simulink model "controllerSharedMem"  (Simulink 8.0)
settings: Solver=FixedStepDiscrete  StartTime=0.0  StopTime=inf  RelTol=1e-3
InitFcn:
  | initSharedMem;
values from neighbouring files (symbols this model uses):
  k = [  10    0.1   2 ... (first row only)    [initRov14.m]    (also in initSharedMem.m = [ 20    5   15)
  kw = block.InputPort(6).Data    [desiredForceComputation.m]    (also in initBalancingControllerWithHandControl.m = 5; initSharedMem.m = 1; initTorqueBalancing.m = 4; initTorqueBalancingWithNonlinearImpedences.m = 1)
  nc = 12    [initCompleteForceControlSim.m]    (also in initPartialForceControl.m = 6; initPartialForceControlSim.m = 6; initSharedMem.m)
  nj = 25    [initCompleteForceControlSim.m]    (also in initMonitor.m; initMonitorSim.m; initPartialForceControl.m; initPartialForceControlSim.m)
undefined symbols (not defined in the file or in its folder): DiscIntNeverNeededParam
libraries: WBCLibrary x17, simulink x3, dspsigops x3
settings Model: Creator=daniele  LastModifiedBy=makaveli
settings DebuggingCC: FcnCallInpInsideContextMsg=EnableAllAsWarning
settings GRTTargetCC: CombineOutputUpdateFcns=off  GRTInterface=on

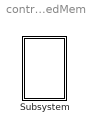
== system controllerSharedMem ==
  Subsystem : Subsystem  mask{robotName='icubGazeboSim', Ts=0.01, localName='dynamicBalancing'}
      mask prompts: robotName "robot name"; localName "module name"

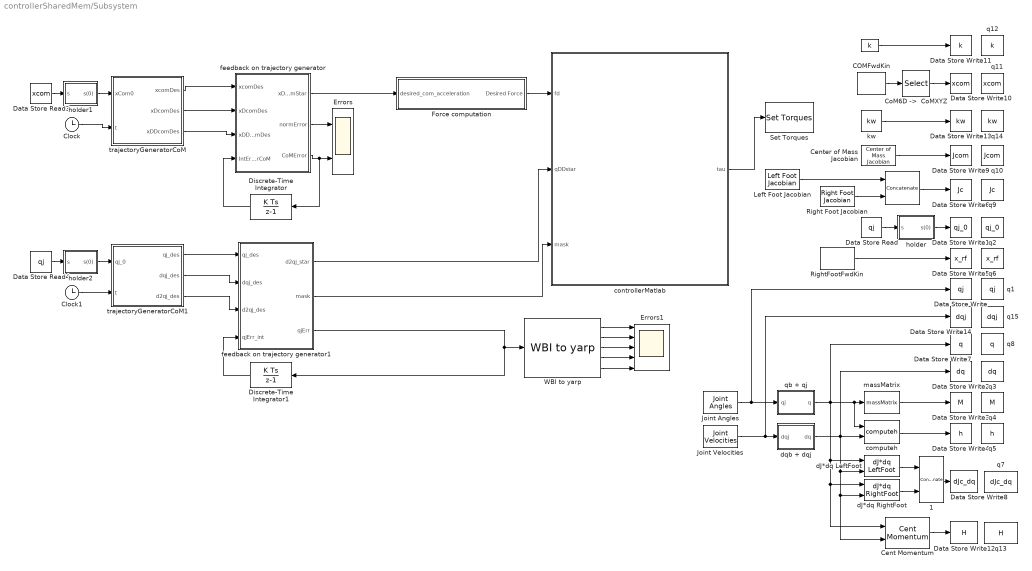
== system controllerSharedMem/Subsystem ==
  "    " : Constant  Value=k
  " " : Concatenate  Mode=Multidimensional array
  " 1" : Concatenate  Mode=Multidimensional array
  "COMFwdKin " : WBCLibrary/wholeBodyModel/Forward Kinematics/COMFwdKin   robotName=robotName  localName=localName
  Cent Momentum : WBCLibrary/wholeBodyModel/Dynamics/Cent Momentum  robotName=robotName  localName=localName
  Center of Mass Jacobian : WBCLibrary/wholeBodyModel/Jacobians/Center of Mass Jacobian  robotName=robotName  localName=localName
  Clock : Clock
  Clock1 : Clock
  "CoM6D ->  CoMXYZ" : Selector  InputPortWidth=7  IndexOptions=Index vector (dialog)  Indices=[1 2 3]  OutputSizes=1
  Data Store Read : DataStoreRead  DataStoreName=qj
  Data Store Read3 : DataStoreRead  DataStoreName=xcom
  Data Store Read4 : DataStoreRead  DataStoreName=qj
  Data Store Write : DataStoreWrite  Priority=-1  DataStoreName=qj
  Data Store Write1 : DataStoreWrite  Priority=-1  DataStoreName=qj_0
  Data Store Write10 : DataStoreWrite  Priority=-1  DataStoreName=xcom
  Data Store Write11 : DataStoreWrite  Priority=-1  DataStoreName=k
  Data Store Write12 : DataStoreWrite  Priority=-1  DataStoreName=H
  Data Store Write13 : DataStoreWrite  Priority=-1  DataStoreName=kw
  Data Store Write14 : DataStoreWrite  Priority=-1  DataStoreName=dqj
  Data Store Write2 : DataStoreWrite  Priority=-1  DataStoreName=dq
  Data Store Write3 : DataStoreWrite  Priority=-1  DataStoreName=M
  Data Store Write4 : DataStoreWrite  Priority=-1  DataStoreName=h
  Data Store Write5 : DataStoreWrite  Priority=-1  DataStoreName=x_rf
  Data Store Write6 : DataStoreWrite  Priority=-1  DataStoreName=Jc
  Data Store Write7 : DataStoreWrite  Priority=-1  DataStoreName=q
  Data Store Write8 : DataStoreWrite  Priority=-1  DataStoreName=dJc_dq
  Data Store Write9 : DataStoreWrite  Priority=-1  DataStoreName=Jcom
  Discrete-Time Integrator : DiscreteIntegrator  InitialCondition=[0;0;0]  SampleTime=Ts  ICPrevOutput=DiscIntNeverNeededParam  ICPrevScaledInput=DiscIntNeverNeededParam
  Discrete-Time Integrator1 : DiscreteIntegrator  InitialCondition=zeros(nj,1)  SampleTime=Ts  ICPrevOutput=DiscIntNeverNeededParam  ICPrevScaledInput=DiscIntNeverNeededParam
  Errors : Scope  NumInputPorts=2
      settings: TimeRange=70  YMin=0~-0.025  YMax=0.0325~0.0325  SaveName=ScopeData6
  Errors1 : Scope  NumInputPorts=5
      settings: TimeRange=70  YMin=-0.2~-0.1~-0.075~-0.25~-0.2  YMax=0.25~0.075~0.1~0.25~0.25
  Force computation : Subsystem
  Joint Angles : WBCLibrary/wholeBodyStates/Joint Angles  robotName=robotName  localName=localName
  Joint Velocities : WBCLibrary/wholeBodyStates/Joint Velocities  robotName=robotName  localName=localName
  Left Foot Jacobian : WBCLibrary/wholeBodyModel/Jacobians/Left Foot Jacobian  robotName=robotName  localName=localName
  Right Foot Jacobian : WBCLibrary/wholeBodyModel/Jacobians/Right Foot Jacobian  robotName=robotName  localName=localName
  RightFootFwdKin : WBCLibrary/wholeBodyModel/Forward Kinematics/RightFootFwdKin  robotName=robotName  localName=localName
  Set Torques : WBCLibrary/wholeBodyActuators/Set Torques  val=6  robotName=robotName  localName=localName
  WBI to yarp : WBCLibrary/Utilities/WBI to yarp
  computeh : WBCLibrary/wholeBodyModel/Dynamics/computeh  val=7  robotname=robotName  localname=localName
  controllerMatlab : MATLAB Function  TreatAsAtomicUnit=on
  dJ*dq LeftFoot : WBCLibrary/wholeBodyModel/Dynamics/dJ*dq LeftFoot  val=9  robotName=robotName  localName=localName
  dJ*dq RightFoot : WBCLibrary/wholeBodyModel/Dynamics/dJ*dq RightFoot  val=9  robotName=robotName  localName=localName
  dqb + dqj : Subsystem
  feedback on trajectory generator : MATLAB Function  TreatAsAtomicUnit=on
  feedback on trajectory generator1 : MATLAB Function  TreatAsAtomicUnit=on
  holder : Subsystem
  holder1 : Subsystem
  holder2 : Subsystem
  kw : Constant  Value=kw
  massMatrix : WBCLibrary/wholeBodyModel/Dynamics/massMatrix  val=8  robotname=robotName  localname=localName
  q1 : DataStoreMemory  Priority=-1  DataStoreName=qj  ReadBeforeWriteMsg=warning  WriteAfterWriteMsg=warning  WriteAfterReadMsg=warning  InitialValue=zeros(nj,1)  VectorParams1D=off  OutDataTypeStr=double
  q10 : DataStoreMemory  Priority=-1  DataStoreName=Jcom  ReadBeforeWriteMsg=warning  WriteAfterWriteMsg=warning  WriteAfterReadMsg=warning  InitialValue=zeros(6,nj+6)  VectorParams1D=off  OutDataTypeStr=double
  q11 : DataStoreMemory  Priority=-1  DataStoreName=xcom  ReadBeforeWriteMsg=warning  WriteAfterWriteMsg=warning  WriteAfterReadMsg=warning  InitialValue=zeros(3,1)  VectorParams1D=off  OutDataTypeStr=double
  q12 : DataStoreMemory  Priority=-1  DataStoreName=k  ReadBeforeWriteMsg=warning  WriteAfterWriteMsg=warning  WriteAfterReadMsg=warning  InitialValue=k  VectorParams1D=off  OutDataTypeStr=double
  q13 : DataStoreMemory  Priority=-1  DataStoreName=H  ReadBeforeWriteMsg=warning  WriteAfterWriteMsg=warning  WriteAfterReadMsg=warning  InitialValue=zeros(6,1)  VectorParams1D=off  OutDataTypeStr=double
  q14 : DataStoreMemory  Priority=-1  DataStoreName=kw  ReadBeforeWriteMsg=warning  WriteAfterWriteMsg=warning  WriteAfterReadMsg=warning  InitialValue=kw  VectorParams1D=off  OutDataTypeStr=double
  q15 : DataStoreMemory  Priority=-1  DataStoreName=dqj  ReadBeforeWriteMsg=warning  WriteAfterWriteMsg=warning  WriteAfterReadMsg=warning  InitialValue=zeros(nj,1)  VectorParams1D=off  OutDataTypeStr=double
  q2 : DataStoreMemory  Priority=-1  DataStoreName=qj_0  ReadBeforeWriteMsg=warning  WriteAfterWriteMsg=warning  WriteAfterReadMsg=warning  InitialValue=zeros(nj,1)  VectorParams1D=off  OutDataTypeStr=double
  q3 : DataStoreMemory  Priority=-1  DataStoreName=dq  ReadBeforeWriteMsg=warning  WriteAfterWriteMsg=warning  WriteAfterReadMsg=warning  InitialValue=zeros(nj+6,1)  VectorParams1D=off  OutDataTypeStr=double
  q4 : DataStoreMemory  Priority=-1  DataStoreName=M  ReadBeforeWriteMsg=warning  WriteAfterWriteMsg=warning  WriteAfterReadMsg=warning  InitialValue=zeros(nj+6,nj+6)  VectorParams1D=off  OutDataTypeStr=double
  q5 : DataStoreMemory  Priority=-1  DataStoreName=h  ReadBeforeWriteMsg=warning  WriteAfterWriteMsg=warning  WriteAfterReadMsg=warning  InitialValue=zeros(nj+6,1)  VectorParams1D=off  OutDataTypeStr=double
  q6 : DataStoreMemory  Priority=-1  DataStoreName=x_rf  ReadBeforeWriteMsg=warning  WriteAfterWriteMsg=warning  WriteAfterReadMsg=warning  InitialValue=zeros(7,1)  VectorParams1D=off  OutDataTypeStr=double
  q7 : DataStoreMemory  Priority=-1  DataStoreName=dJc_dq  ReadBeforeWriteMsg=warning  WriteAfterWriteMsg=warning  WriteAfterReadMsg=warning  InitialValue=zeros(nc,1)  VectorParams1D=off  OutDataTypeStr=double
  q8 : DataStoreMemory  Priority=-1  DataStoreName=q  ReadBeforeWriteMsg=warning  WriteAfterWriteMsg=warning  WriteAfterReadMsg=warning  InitialValue=zeros(nj+16,1)  VectorParams1D=off  OutDataTypeStr=double
  q9 : DataStoreMemory  Priority=-1  DataStoreName=Jc  ReadBeforeWriteMsg=warning  WriteAfterWriteMsg=warning  WriteAfterReadMsg=warning  InitialValue=zeros(nc,nj+6)  VectorParams1D=off  OutDataTypeStr=double
  qb + qj : Subsystem
  trajectoryGeneratorCoM : MATLAB Function  TreatAsAtomicUnit=on
  trajectoryGeneratorCoM1 : MATLAB Function  TreatAsAtomicUnit=on
  wires:
  Left Foot Jacobian/1 -> " "/1
  Right Foot Jacobian/1 -> " "/2
  qb + qj/1(q) -> massMatrix/1, computeh/1, dJ*dq LeftFoot/1, Cent Momentum/1, dJ*dq RightFoot/1, Data Store Write7/1
  dqb + dqj/1(dq) -> computeh/2, dJ*dq LeftFoot/2, Cent Momentum/2, dJ*dq RightFoot/2, Data Store Write2/1
  Data Store Read/1 -> holder/1(s)
  holder/1(s(0)) -> Data Store Write1/1
  massMatrix/1 -> Data Store Write3/1
  computeh/1 -> Data Store Write4/1
  Joint Velocities/1 -> dqb + dqj/1(dqj), Data Store Write14/1
  RightFootFwdKin/1 -> Data Store Write5/1
  " "/1 -> Data Store Write6/1
  "    "/1 -> Data Store Write11/1
  Center of Mass Jacobian/1 -> Data Store Write9/1
  "COMFwdKin "/1 -> "CoM6D ->  CoMXYZ"/1
  "CoM6D ->  CoMXYZ"/1 -> Data Store Write10/1
  Clock/1 -> trajectoryGeneratorCoM/2(t)
  holder1/1(s(0)) -> trajectoryGeneratorCoM/1(xCom0)
  dJ*dq LeftFoot/1 -> " 1"/1
  dJ*dq RightFoot/1 -> " 1"/2
  " 1"/1 -> Data Store Write8/1
  Cent Momentum/1 -> Data Store Write12/1
  kw/1 -> Data Store Write13/1
  controllerMatlab/1(tau) -> Set Torques/1
  Data Store Read3/1 -> holder1/1(s)
  trajectoryGeneratorCoM/1(xcomDes) -> feedback on trajectory generator/1(xcomDes)
  trajectoryGeneratorCoM/2(xDcomDes) -> feedback on trajectory generator/2(xDcomDes)
  trajectoryGeneratorCoM/3(xDDcomDes) -> feedback on trajectory generator/3(xDDcomDes)
  Discrete-Time Integrator/1 -> feedback on trajectory generator/4(IntErrorCoM)
  feedback on trajectory generator/2(normError) -> Errors/1
  Clock1/1 -> trajectoryGeneratorCoM1/2(t)
  holder2/1(s(0)) -> trajectoryGeneratorCoM1/1(qj_0)
  Data Store Read4/1 -> holder2/1(s)
  trajectoryGeneratorCoM1/1(qj_des) -> feedback on trajectory generator1/1(qj_des)
  trajectoryGeneratorCoM1/2(dqj_des) -> feedback on trajectory generator1/2(dqj_des)
  trajectoryGeneratorCoM1/3(d2qj_des) -> feedback on trajectory generator1/3(d2qj_des)
  Discrete-Time Integrator1/1 -> feedback on trajectory generator1/4(qjErr_int)
  Joint Angles/1 -> qb + qj/1(qj), Data Store Write/1
  feedback on trajectory generator/3(CoMError) -> Errors/2, Discrete-Time Integrator/1
  feedback on trajectory generator1/1(d2qj_star) -> controllerMatlab/2(qDDstar)
  WBI to yarp/1 -> Errors1/1
  WBI to yarp/2 -> Errors1/2
  WBI to yarp/3 -> Errors1/3
  WBI to yarp/4 -> Errors1/4
  WBI to yarp/5 -> Errors1/5
  feedback on trajectory generator1/3(qjErr) -> WBI to yarp/1, Discrete-Time Integrator1/1
  feedback on trajectory generator1/2(mask) -> controllerMatlab/3(mask)
  feedback on trajectory generator/1(xDDcomStar) -> Force computation/1(desired_com_acceleration)
  Force computation/1(Desired Force) -> controllerMatlab/1(fd)

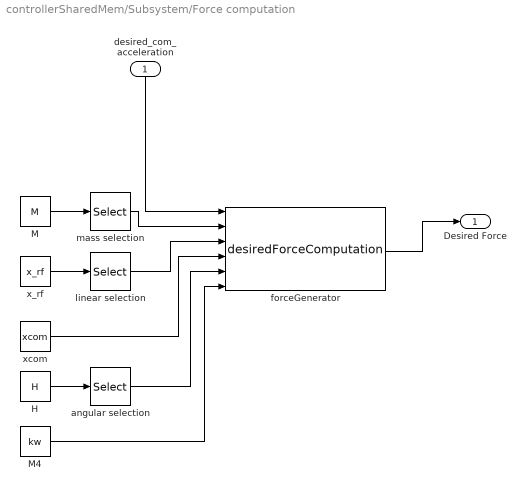
== system controllerSharedMem/Subsystem/Force computation ==
  desired_com_acceleration : Inport
  H : DataStoreRead  DataStoreName=H
  M : DataStoreRead  DataStoreName=M
  M4 : DataStoreRead  DataStoreName=kw
  angular selection : Selector  InputPortWidth=6  IndexOptions=Index vector (dialog)  Indices=[4:6]  OutputSizes=1
  forceGenerator : M-S-Function  FunctionName=desiredForceComputation
  linear selection : Selector  InputPortWidth=7  IndexOptions=Index vector (dialog)  Indices=[1:3]  OutputSizes=1
  mass selection : Selector  NumberOfDimensions=2  InputPortWidth=3  IndexOptions=Index vector (dialog),Index vector (dialog)  Indices=1,1  OutputSizes=1,1
  x_rf : DataStoreRead  DataStoreName=x_rf
  xcom : DataStoreRead  DataStoreName=xcom
  Desired Force : Outport
  wires:
  forceGenerator/1 -> Desired Force/1
  mass selection/1 -> forceGenerator/2
  x_rf/1 -> linear selection/1
  xcom/1 -> forceGenerator/4
  desired_com_acceleration/1 -> forceGenerator/1
  M/1 -> mass selection/1
  linear selection/1 -> forceGenerator/3
  angular selection/1 -> forceGenerator/5
  H/1 -> angular selection/1
  M4/1 -> forceGenerator/6

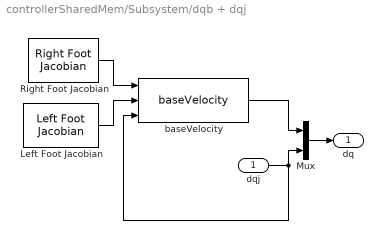
== system controllerSharedMem/Subsystem/dqb + dqj ==
  dqj : Inport
  Left Foot Jacobian : WBCLibrary/wholeBodyModel/Jacobians/Left Foot Jacobian  robotName=robotName  localName=localName
  Mux : Mux  Inputs=2
  Right Foot Jacobian : WBCLibrary/wholeBodyModel/Jacobians/Right Foot Jacobian  robotName=robotName  localName=localName
  baseVelocity : WBCLibrary/Utilities/baseVelocity
  dq : Outport
  wires:
  Left Foot Jacobian/1 -> baseVelocity/2
  Right Foot Jacobian/1 -> baseVelocity/1
  baseVelocity/1 -> Mux/1
  dqj/1 -> baseVelocity/3, Mux/2
  Mux/1 -> dq/1

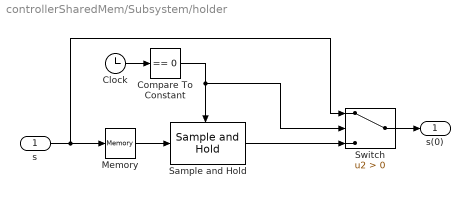
== system controllerSharedMem/Subsystem/holder ==
  s : Inport
  Clock : Clock
  Compare To Constant : simulink/Logic and Bit Operations/Compare To Constant  relop===  const=0  OutDataTypeStr=boolean
  Memory : Memory
  Sample and Hold : dspsigops/Sample and Hold  trig=Falling edge  initCond=0  latchinput=off
  Switch : Switch  Criteria=u2 > Threshold
  s(0) : Outport
  wires:
  s/1 -> Switch/1, Memory/1
  Clock/1 -> Compare To Constant/1
  Compare To Constant/1 -> Sample and Hold/Trigger, Switch/2
  Sample and Hold/1 -> Switch/3
  Switch/1 -> s(0)/1
  Memory/1 -> Sample and Hold/1

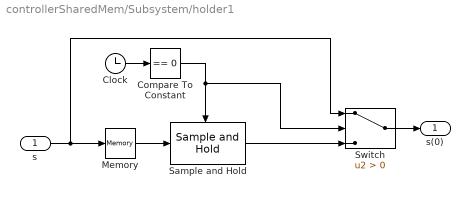
== system controllerSharedMem/Subsystem/holder1 ==
  s : Inport
  Clock : Clock
  Compare To Constant : simulink/Logic and Bit Operations/Compare To Constant  relop===  const=0  OutDataTypeStr=boolean
  Memory : Memory
  Sample and Hold : dspsigops/Sample and Hold  trig=Falling edge  initCond=0  latchinput=off
  Switch : Switch  Criteria=u2 > Threshold
  s(0) : Outport
  wires:
  s/1 -> Switch/1, Memory/1
  Clock/1 -> Compare To Constant/1
  Compare To Constant/1 -> Sample and Hold/Trigger, Switch/2
  Sample and Hold/1 -> Switch/3
  Switch/1 -> s(0)/1
  Memory/1 -> Sample and Hold/1

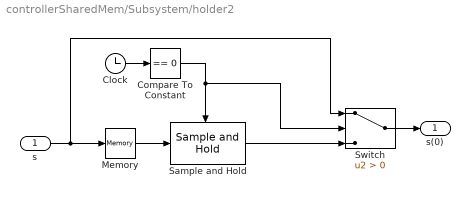
== system controllerSharedMem/Subsystem/holder2 ==
  s : Inport
  Clock : Clock
  Compare To Constant : simulink/Logic and Bit Operations/Compare To Constant  relop===  const=0  OutDataTypeStr=boolean
  Memory : Memory
  Sample and Hold : dspsigops/Sample and Hold  trig=Falling edge  initCond=0  latchinput=off
  Switch : Switch  Criteria=u2 > Threshold
  s(0) : Outport
  wires:
  s/1 -> Switch/1, Memory/1
  Clock/1 -> Compare To Constant/1
  Compare To Constant/1 -> Sample and Hold/Trigger, Switch/2
  Sample and Hold/1 -> Switch/3
  Switch/1 -> s(0)/1
  Memory/1 -> Sample and Hold/1

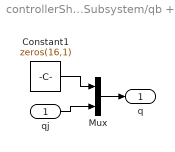
== system controllerSharedMem/Subsystem/qb + qj ==
  qj : Inport
  Constant1 : Constant  Value=zeros(16,1)
  Mux : Mux  Inputs=2
  q : Outport
  wires:
  Mux/1 -> q/1
  Constant1/1 -> Mux/1
  qj/1 -> Mux/2

== matlab function Subsystem/trajectoryGeneratorCoM ==
  data: xcomDes output double; xCom0 input double; t input double; Jcom data_store_memory double; xDcomDes output double; xDDcomDes output double; dq data_store_memory double; k data_store_memory double
function [xcomDes, xDcomDes, xDDcomDes]  = trajGen(xCom0,t)
%#codegen


e3 = [0;1;0];
A = 0.1;
f = 0.1;
t = t*0.8;
% xcomDes    = [xCom0(1:2); (1/A-1)*A*xCom0(3)] + A*xCom0(3)*cos(2*pi*f*t)*e3;
% xDcomDes   = -xCom0(3)*A*2*pi*f*sin(2*pi*f*t)*e3;
% xDDcomDes  = -xCom0(3)*A*(2*pi*f)^2*cos(2*pi*f*t)*e3;

xcomDes    = xCom0 + A*sin(2*pi*f*t)*e3;
xDcomDes   =         A*2*pi*f*cos(2*pi*f*t)*e3;
xDDcomDes  =        -A*(2*pi*f)^2*sin(2*pi*f*t)*e3;

== matlab function Subsystem/controllerMatlab ==
  data: qj data_store_memory double; qj_0 data_store_memory double; dq data_store_memory double; M data_store_memory double; h data_store_memory double; x_rf data_store_memory double; Jc data_store_memory double; tau output double; xcom data_store_memory double; fd input double; H data_store_memory double; dJc_dq data_store_memory double; k data_store_memory double; kw data_store_memory double; qDDstar input double; mask input double
function tau  = computeTau(fd, qDDstar, mask)
%#codegen

global qj dq qj_0 
global M h Jc dJc_dq
global k

nt = 25;

PINV_TOL = 1e-5;
g        = 9.81;

DL = 25-nt;            %DeltaIndexOnlyLegs

if DL ~= 0
   Jcr = [Jc(:,1:6),Jc(:,7 + DL:end)]; 
else
   Jcr = Jc; 
end

m     = M(1,1);
Mb    = M(1:6,1:6);
MbInv = inv(Mb);
Mbj   = M(1:6,7 + DL :end); 
Mj    = M(7 + DL :end,7 + DL:end);
U     = [eye(6) , zeros(6,nt)];
Jcb   = Jcr*U';
SBar  = [  -MbInv*Mbj 
           eye(nt)      ];
NjInv = Mj - Mbj'*MbInv*Mbj;


JcSBar     = Jcr*SBar;
JcSBarPinv = pinv(JcSBar, PINV_TOL);

% Definition of reference accelerations for CoM and Joints that ensure
% stabilization of desired trajectories xDcomDes and qDes 

if DL ~= 0
   q_star = qDDstar(DL+1:end); 
else
   q_star = qDDstar;
    
end


LambdaStar = JcSBarPinv*(Jcb*MbInv*(h(1:6) - Jcb'*fd) - dJc_dq);

NP0 = eye(nt) - JcSBarPinv*JcSBar;

LambdaStar = LambdaStar + NP0 * q_star;

tauLegs = - JcSBar'*fd + NjInv*LambdaStar + SBar'*[h(1:6);h(DL + 7:end)];

tau = h(7:end) - k(3,1)*(qj - qj_0) - k(3,3)*dq(7:end);   
tau(mask) = tauLegs(mask);

== matlab function Subsystem/feedback on trajectory generator ==
  data: xDDcomStar output double; normError output double; xcomDes input double; xDcomDes input double; xDDcomDes input double; IntErrorCoM input double; Jcom data_store_memory double; CoMError output double; dq data_store_memory double; k data_store_memory double; xcom data_store_memory double
function [xDDcomStar, normError, CoMError]  = fcn(xcomDes, xDcomDes, xDDcomDes, IntErrorCoM)
%#codegen

global Jcom dq k xcom

xDcom      = Jcom(1:3,:)*dq;
xDDcomStar = xDDcomDes - k(1,1)*(xcom - xcomDes) - k(1,2)*IntErrorCoM - k(1,3)*(xDcom - xDcomDes)  ;

CoMError    = xcom - xcomDes;
normError   = norm(CoMError);

== matlab function Subsystem/feedback on trajectory generator1 ==
  data: d2qj_star output double; mask output double; qj_des input double; dqj_des input double; d2qj_des input double; qjErr output double; Jcom data_store_memory double; k data_store_memory double; qjErr_int input double; qj data_store_memory double; dqj data_store_memory double
function [d2qj_star, mask, qjErr]   = fcn(qj_des, dqj_des, d2qj_des, qjErr_int)
%#codegen

global k qj dqj

d2qj_star   = d2qj_des - k(2,1)*(qj - qj_des) - k(2,2)*qjErr_int- k(2,3)*(dqj - dqj_des);

qjErr = qj - qj_des;

mask = (abs(qjErr) < 0.2);

== matlab function Subsystem/trajectoryGeneratorCoM1 ==
  data: qj_des output double; qj_0 input double; t input double; Jcom data_store_memory double; dqj_des output double; d2qj_des output double; dq data_store_memory double; k data_store_memory double
function [qj_des, dqj_des, d2qj_des]  = trajGen(qj_0,t)
%#codegen


qj_des    = qj_0;
dqj_des   = zeros(size(qj_0));
d2qj_des  = zeros(size(qj_0));
